simulink subsystem "calcErrorInnerLoop"  (R2026a)
settings: Solver=VariableStepAuto
settings Model: Creator=maxhu  LastModifiedBy=maxhu

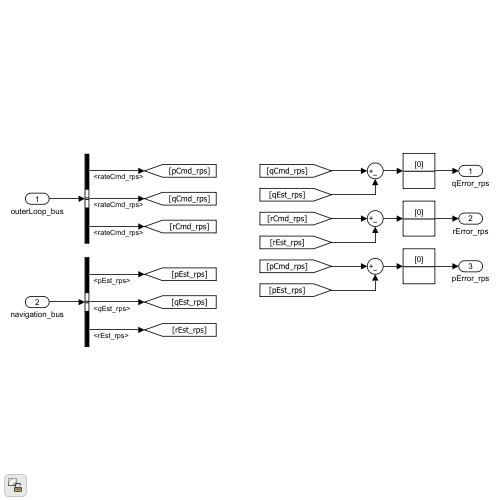
[thumbnail: Simulink's stored preview of the top-level diagram]
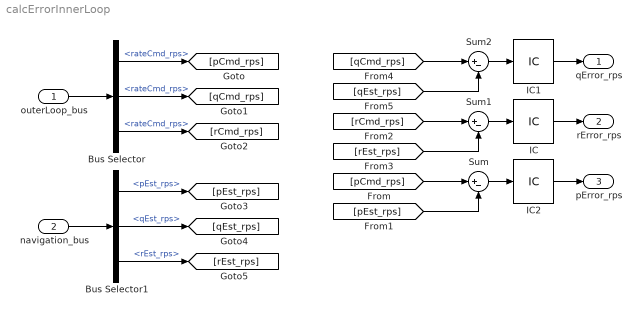
== system calcErrorInnerLoop ==
  outerLoop_bus : Inport
  navigation_bus : Inport  Port=2
  Bus Selector : BusSelector  OutputSignals=rollOuterLoop_bus.rateCmd_rps,pitchOuterLoop_bus.rateCmd_rps,yawOuterLoop_bus.rateCmd_rps
  Bus Selector1 : BusSelector  OutputSignals=pEst_rps,qEst_rps,rEst_rps
  IC : InitialCondition  Value=0
  IC1 : InitialCondition  Value=0
  IC2 : InitialCondition  Value=0
  Sum : Sum  Inputs=|+-
  Sum1 : Sum  Inputs=|+-
  Sum2 : Sum  Inputs=|+-
  qError_rps : Outport
  rError_rps : Outport  Port=2
  pError_rps : Outport  Port=3
  wires:
  Bus Selector1/1 -> [pEst_rps]  "<pEst_rps>"
  Bus Selector1/2 -> [qEst_rps]  "<qEst_rps>"
  Bus Selector1/3 -> [rEst_rps]  "<rEst_rps>"
  navigation_bus/1 -> Bus Selector1/1
  [qCmd_rps] -> Sum2/1
  [qEst_rps] -> Sum2/2
  [pCmd_rps] -> Sum/1
  Sum2/1 -> IC1/1
  Sum1/1 -> IC/1
  [pEst_rps] -> Sum/2
  Bus Selector/1 -> [pCmd_rps]  "<rateCmd_rps>"
  [rEst_rps] -> Sum1/2
  [rCmd_rps] -> Sum1/1
  outerLoop_bus/1 -> Bus Selector/1
  Sum/1 -> IC2/1
  Bus Selector/2 -> [qCmd_rps]  "<rateCmd_rps>"
  IC1/1 -> qError_rps/1
  IC/1 -> rError_rps/1
  IC2/1 -> pError_rps/1
  Bus Selector/3 -> [rCmd_rps]  "<rateCmd_rps>"
